simulink model "smd"  (R2014a)
settings: Solver=ode45  StartTime=0.0  StopTime=0.1  RelTol=1e-3
values from neighbouring files (symbols this model uses):
  C = 1*10^-6    (= 1e-06)    [rlc.m]
  L = 1    [rlc.m]
  R = 4.7*10^3    (= 4700)    [rlc.m]
  V = 5    [rlc.m]
settings Model: Creator=Diana  LastModifiedBy=Diana

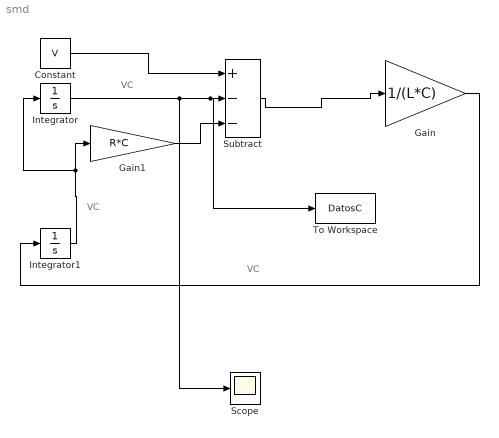
== system smd ==
  note: VC
  note: VC
  note: VC
  Constant : Constant  Value=V
  Gain : Gain  Gain=1/(L*C)
  Gain1 : Gain  Gain=R*C
  Integrator : Integrator
  Integrator1 : Integrator
  Scope : Scope
  Subtract : Sum  Inputs=+--
  To Workspace : ToWorkspace  VariableName=DatosC  SaveFormat=Timeseries  SampleTime=-1
  wires:
  Subtract/1 -> Gain/1
  Constant/1 -> Subtract/1
  Integrator/1 -> Scope/1, To Workspace/1, Subtract/2
  Gain1/1 -> Subtract/3
  Gain/1 -> Integrator1/1
  Integrator1/1 -> Integrator/1, Gain1/1
